simulink model "SEPIC_PV_system_MPPT_Alogrithms_BATTERY"  (R2025a)
settings: Solver=FixedStepAuto  StartTime=0.0  StopTime=1  FixedStep=1e-7  RelTol=1e-3
undefined symbols (not defined in the file): Ion, Lithium, sigbuilder_block
libraries: spsSeriesRLCBranchLib x6, spsCurrentMeasurementLib x5, spsVoltageMeasurementLib x3, spsGroundLib x2, spsBatteryLib x1, spsDiodeLib x1, spsMosfetLib x1, spsPVArrayLib x1, simulink x1, simulink_extras x1, sps_lib x1
settings Model: Creator=gamezebra  LastModifiedBy=gamezebra

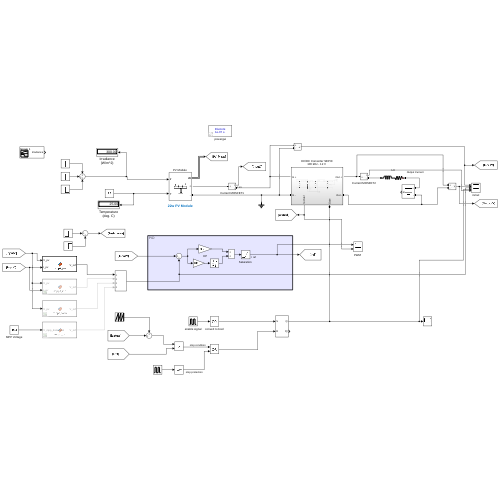
[thumbnail: Simulink's stored preview of the top-level diagram]
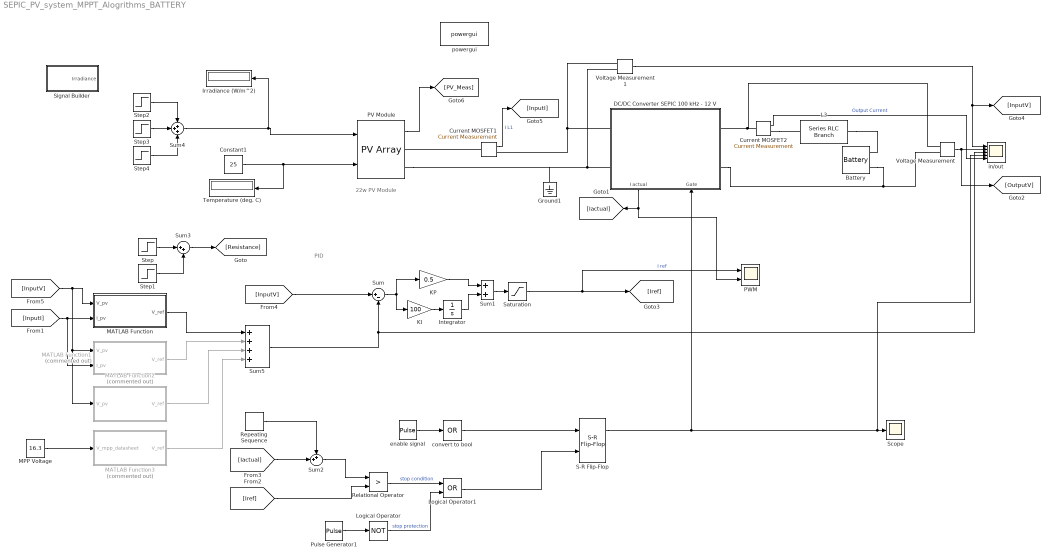
== system SEPIC_PV_system_MPPT_Alogrithms_BATTERY ==
  note: PID
  note: 22w PV Module
  Battery : spsBatteryLib/Battery  BatType=Lithium-Ion  NomV=10.8  NomQ=1  SOC=3  Batt_Tr=30  PresetModel=on  MaxQ=1  MinV=8.1  FullV=12.5711  Dis_rate=0.43478  R=0.108  Normal_OP=0.90435  expZone="[11.6682    0.0491304]"
  Constant1 : Constant  Value=25
  Current MOSFET1 : spsCurrentMeasurementLib/Current Measurement  PhasorSimulation=off  OutputType=Complex  PSBequivalent=0
  Current MOSFET2 : spsCurrentMeasurementLib/Current Measurement  PhasorSimulation=off  OutputType=Complex  PSBequivalent=0
  "DC/DC Converter SEPIC 100 kHz - 12 V " : Subsystem
      settings: PortSchema="{\"entries\":[{\"content\":{\"sides\":[{\"content\":{\"connectorIds\":[\"LConn1\",\"LConn2\"]},\"type\":\"ConnectorPlacement.EquallySpacedRectSide\",\"uuid\":\"91feb529-5820-4edf-8d0e-1c637fed9421\"},{\"content\":{\"connectorIds\":[\"RConn1\",\"RConn2\"],\"side\":\"RIGHT\"},\"type\":\"ConnectorPlacement.EquallySpacedRectSide\",\"uuid\":\"b4099113-c0ef-4c50-8083-88b14b98cc04\"},{\"content\":{\"side\":\"TOP\"},\"type\":\"ConnectorPlacement.EquallySpacedRectSide\",\"uuid\":\"250c6351-2de3-43d7-b6c9-3c3ed0452184\"},{\"content\":{\"connectorIds\":[\"Out1\",\"In1\"],\"side\":\"BOTTOM\"},\"type\":\"ConnectorPlacement.EquallySpacedRectSide\",\"uuid\":\"484af620-bbf2-4328-991e-a08b15b59058\"}]},\"type\":\"ConnectorPlacement.EquallySpacedConnector\",\"uuid\":\"7041a545-1967-46d5-8643-e26f6c990daf\"}],\"packageUris\":[\"http://schema.mathworks.com/mf0/Connector/R2020b\"],\"version\":\"1.0\"}"
  Ground1 : spsGroundLib/Ground  LConnTagsString=a
  Integrator : Integrator  LimitOutput=on  UpperSaturationLimit=8  LowerSaturationLimit=0
  Irradiance (W/m^2) : Display
      settings: Format=bank  Decimation=1000
  KI : Gain  Gain=100
  KP : Gain  Gain=0.5
  L3 : spsSeriesRLCBranchLib/Series RLC Branch  LConnTagsString=__new0  RConnTagsString=__new0  BranchType=RL  Resistance=0.1  Inductance=5e-6  SetiL0=off  InitialCurrent=0  Capacitance=1e-6  Setx0=off  InitialVoltage=0  Measurements=None
  Logical Operator : Logic  Operator=NOT  AllPortsSameDT=off  OutDataTypeStr=boolean
  Logical Operator1 : Logic  Operator=OR  AllPortsSameDT=off  OutDataTypeStr=boolean
  MATLAB Function : MATLAB Function  TreatAsAtomicUnit=on
  MATLAB Function1 : MATLAB Function  Commented=on  TreatAsAtomicUnit=on
  MATLAB Function2 : MATLAB Function  Commented=on  TreatAsAtomicUnit=on
  MATLAB Function3 : MATLAB Function  Commented=on  TreatAsAtomicUnit=on
  MPP Voltage : Constant  Value=16.3
  "PV Module " : spsPVArrayLib/PV Array  Npar=1  Nser=1  PlotType=one module @ 25 deg.C & specified irradiances  S_vec="[ 1000  500  200 ]"  Temp_C_vec=25  ModuleName=User-defined  PlotWhenSelected=off  Pm=21.6138  Ncell=30  Voc=17.76  Isc=1.5  Vm=16.3  Im=1.326  beta_Voc_pc=-0.37  alpha_Isc_pc=0.07  beta_Voc=-0.065712  alpha_Isc=0.00105  IL=1.5  I0=2.021e-11  nI=1.0007  Rsh=187.3567  Rs=0.40236  RobustModel=off  RobustCellTemperature=313.3991  BAL=on  Tc=1e-6  Tfilter=5e-5
  "PWM " : Scope  NumInputPorts=2
      settings: Title=PWM  ActiveDisplayYMinimum=3.3246670438564179  ActiveDisplayYMaximum=8.2208811739016561  YLabel=Amplitudo
  Pulse Generator1 : DiscretePulseGenerator  PulseType=Time based  Period=10e-6  PulseWidth=90
  Relational Operator : RelationalOperator  Operator=>  OutDataTypeStr=boolean  RndMeth=Simplest  InputSameDT=off
  Repeating Sequence : simulink/Sources/Repeating Sequence  rep_seq_t=[0 10e-6]  rep_seq_y=[0 2]
  S-R Flip-Flop : simulink_extras/Flip Flops/S-R Flip-Flop  initial_condition=0
  "Saturation " : Saturate  UpperLimit=8  LowerLimit=0
  Scope : Scope
      settings: ActiveDisplayYMinimum=-0.12499999999999997  ActiveDisplayYMaximum=1.125  DataLoggingVariableName=ScopeData2
  Signal Builder : Subsystem  Tag=STV Subsys  LoadFcn=sigbuilder_block('load');  StartFcn=sigbuilder_block('start');  StopFcn=sigbuilder_block('stop');  ClipboardFcn=sigbuilder_block('clipboard');  mask(Sigbuilder block){tuvar=[0:10]}
      mask help: Simulink:masks:SigbuilderBlock_MD
      mask init:
      | if ~strcmp(get_param(bdroot(gcbh),'SimulationStatus'),'stopped') tuvar = sigbuilder_block('maskInit'); end
      settings: CopyFcn=sigbuilder_block('copy');  DeleteFcn=sigbuilder_block('delete');  ModelCloseFcn=sigbuilder_block('modelClose');  PreSaveFcn=sigbuilder_block('preSave');  PauseFcn=sigbuilder_block('pause');  ContinueFcn=sigbuilder_block('continue');  NameChangeFcn=sigbuilder_block('namechange');  OpenFcn=sigbuilder_block('open',[237.75 162.75 783 471.75 ]);  CloseFcn=sigbuilder_block('close');
      mask Display: plot(0, 0, 100, 100,[2, 2, 32, 32, 2], [68, 8, 8, 68, 68],[32, 2], [38, 38], [32, 19, 2],[53, 60, 44], [32, 17, 17, 2],[16, 16, 31, 31]);txt = getActiveGroup(gcbh);text(2, 100, txt,'verticalAlignment', 'top');
  Step : Step  Time=0  After=0  SampleTime=0
  Step1 : Step  Time=0  After=30  SampleTime=0
  Step2 : Step  Time=0.3  Before=1000  After=800  SampleTime=0
  Step3 : Step  Time=0.5  After=-300  SampleTime=0
  Step4 : Step  Time=0.7  After=-200  SampleTime=0
  Sum : Sum  Inputs=|+-
  Sum1 : Sum
  Sum2 : Sum  Inputs=++|
  Sum3 : Sum  Inputs=|++
  Sum4 : Sum  Inputs=+++
  Sum5 : Sum  Inputs=++++
  Temperature (deg. C) : Display
      settings: Format=bank  Decimation=1000
  Voltage Measurement : spsVoltageMeasurementLib/Voltage Measurement  PhasorSimulation=off  OutputType=Complex  PSBequivalent=0
  Voltage Measurement1 : spsVoltageMeasurementLib/Voltage Measurement  PhasorSimulation=off  OutputType=Complex  PSBequivalent=0
  convert to bool : Logic  Operator=OR  Inputs=1  AllPortsSameDT=off  OutDataTypeStr=boolean
  enable signal : DiscretePulseGenerator  PulseType=Time based  Period=10e-6  PulseWidth=5
  in/out : Scope  NumInputPorts=5
      settings: Title=PWM  ActiveDisplayYMinimum=-3.0785426285562241  ActiveDisplayYMaximum=22.486425523480442  YLabel=Amplitudo  DataLoggingVariableName=ScopeData3
  powergui : sps_lib/powergui  Priority=1  SimulationMode=Discrete  SampleTime=1e-7  frequency=60  Iterations=50  frequencyindice=0  Pbase=100e6  ErrMax=1e-4  UnitsV=kV  UnitsW=MW  buscounter=0  FunctionMessages=off  echomessages=off  EnableUseOfTLC=off  CurrentSourceSwitches=off  DisableSnubberDevices=off  DisableRonSwitches=off  DisableVfSwitches=off  DisplayEquations=off  AutomaticDiscreteSolvers=off  SolverType=Tustin/Backward Euler (TBE)  Interpol=off  ExternalGateDelay=off  methode=off  Ts=100  x0status=blocks  SPID=on  SwTol=0  HookPort=off  NonlinearTolerance=1e-4  nMaxIteration=100  ContinueOnMaxIteration=off  RestoreLinks=warning  ResistiveCurrentMeasurement=off  Frange=[0:2:500]  Ylog=off  Xlog=on  ShowGrid=off  save=off  variable=ZData  structure=0  ZoomFFT=off  StartTime=0.0  cycles=1  DisplayStyle=1  fundamental=60  FreqAxis=off  MaxFrequency=1000  frequencyindicesteady=1  RmsSteady=1  display=off
  wires:
  Voltage Measurement1/1 -> in/out/1, [InputV]
  Voltage Measurement/1 -> [OutputV], in/out/2
  Step/1 -> Sum3/1
  Sum1/1 -> "Saturation "/1
  KI/1 -> Integrator/1
  Integrator/1 -> Sum1/2
  KP/1 -> Sum1/1
  Sum/1 -> KI/1, KP/1
  "Saturation "/1 -> "PWM "/1, [Iref]  "I ref"
  [InputV] -> Sum/1
  S-R Flip-Flop/1 -> in/out/4, Scope/1, "DC/DC Converter SEPIC 100 kHz - 12 V "/1(Gate)
  [Iactual] -> Sum2/2
  Pulse Generator1/1 -> Logical Operator/1
  Relational Operator/1 -> Logical Operator1/1  "stop condition"
  Logical Operator/1 -> Logical Operator1/2  "stop protection"
  "DC/DC Converter SEPIC 100 kHz - 12 V "/1(I actual) -> "PWM "/2, [Iactual]
  [Iref] -> Relational Operator/2
  Logical Operator1/1 -> S-R Flip-Flop/2
  enable signal/1 -> convert to bool/1
  convert to bool/1 -> S-R Flip-Flop/1
  Repeating Sequence/1 -> Sum2/1
  Sum2/1 -> Relational Operator/1
  Step1/1 -> Sum3/2
  Sum3/1 -> [Resistance]
  "PV Module "/1 -> [PV_Meas]
  Constant1/1 -> "PV Module "/2, Temperature (deg. C)/1
  Step3/1 -> Sum4/2
  Step2/1 -> Sum4/1
  Step4/1 -> Sum4/3
  Current MOSFET1/1 -> [InputI]  "I L1"
  [InputI] -> MATLAB Function1/2(I_pv), MATLAB Function/2(I_pv)
  [InputV] -> MATLAB Function2/1(V_pv), MATLAB Function1/1(V_pv), MATLAB Function/1(V_pv)
  MATLAB Function/1(V_ref) -> Sum5/1
  Sum4/1 -> Irradiance (W/m^2)/1, "PV Module "/1
  Sum5/1 -> in/out/3, Sum/2
  MATLAB Function1/1(V_ref) -> Sum5/2
  MATLAB Function2/1(V_ref) -> Sum5/3
  MATLAB Function3/1(V_ref) -> Sum5/4
  MPP Voltage/1 -> MATLAB Function3/1(V_mpp_datasheet)
  Current MOSFET2/1 -> in/out/5  "Output Current"
  connections:
  Voltage Measurement1/LConn1 -- Current MOSFET1/RConn1 -- "DC/DC Converter SEPIC 100 kHz - 12 V "/LConn1
  Current MOSFET2/RConn1 -- L3/RConn1
  "DC/DC Converter SEPIC 100 kHz - 12 V "/RConn2 -- Battery/LConn2 -- Voltage Measurement/LConn2
  "DC/DC Converter SEPIC 100 kHz - 12 V "/LConn2 -- Voltage Measurement1/LConn2 -- "PV Module "/RConn2 -- Ground1/LConn1
  Current MOSFET1/LConn1 -- "PV Module "/RConn1
  Voltage Measurement/LConn1 -- Current MOSFET2/LConn1 -- "DC/DC Converter SEPIC 100 kHz - 12 V "/RConn1
  L3/LConn1 -- Battery/LConn1

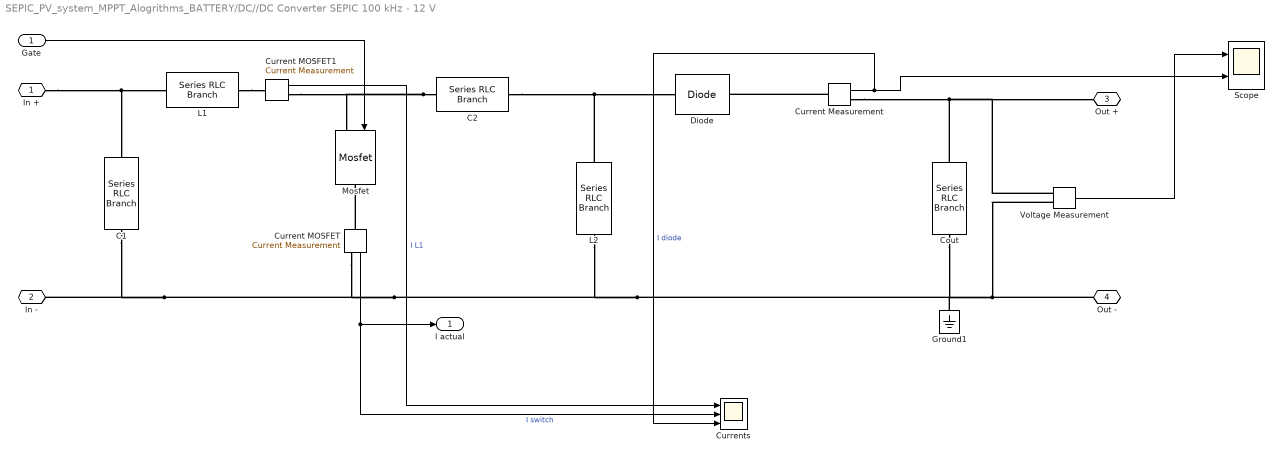
== system SEPIC_PV_system_MPPT_Alogrithms_BATTERY/DC//DC Converter SEPIC 100 kHz - 12 V  ==
  Gate : Inport
  C1 : spsSeriesRLCBranchLib/Series RLC Branch  LConnTagsString=__new0  RConnTagsString=__new0  BranchType=RC  Resistance=0.01  Inductance=1e-3  SetiL0=off  InitialCurrent=0  Capacitance=0.00001  Setx0=on  InitialVoltage=18  Measurements=None
  C2 : spsSeriesRLCBranchLib/Series RLC Branch  LConnTagsString=__new0  RConnTagsString=__new0  BranchType=C  Resistance=1  Inductance=1e-3  SetiL0=off  InitialCurrent=0  Capacitance=0.00001  Setx0=off  InitialVoltage=0  Measurements=None
  Cout : spsSeriesRLCBranchLib/Series RLC Branch  LConnTagsString=__new0  RConnTagsString=__new0  BranchType=RC  Resistance=0.01  Inductance=16.8e-3  SetiL0=off  InitialCurrent=0  Capacitance=0.0001  Setx0=on  InitialVoltage=11.63  Measurements=None
  Current MOSFET : spsCurrentMeasurementLib/Current Measurement  PhasorSimulation=off  OutputType=Complex  PSBequivalent=0
  Current MOSFET1 : spsCurrentMeasurementLib/Current Measurement  PhasorSimulation=off  OutputType=Complex  PSBequivalent=0
  "Current Measurement " : spsCurrentMeasurementLib/Current Measurement  PhasorSimulation=off  OutputType=Complex  PSBequivalent=0
  Currents : Scope  NumInputPorts=3
      settings: ActiveDisplayYMinimum=-2.4566036573506662  ActiveDisplayYMaximum=3.5153800209257291  DataLoggingVariableName=ScopeData4
  "Diode " : spsDiodeLib/Diode  Ron=0.001  Lon=0  Vf=0.5  IC=0  UseSnubber=0  Rs=500  Cs=250e-9  Measurements=off
  Ground1 : spsGroundLib/Ground  LConnTagsString=a
  L1 : spsSeriesRLCBranchLib/Series RLC Branch  LConnTagsString=__new0  RConnTagsString=__new0  BranchType=RL  Resistance=0.2  Inductance=0.0002  SetiL0=off  InitialCurrent=0  Capacitance=1e-6  Setx0=off  InitialVoltage=0  Measurements=None
  L2 : spsSeriesRLCBranchLib/Series RLC Branch  LConnTagsString=__new0  RConnTagsString=__new0  BranchType=RL  Resistance=0.2  Inductance=0.0002  SetiL0=off  InitialCurrent=0  Capacitance=1e-6  Setx0=off  InitialVoltage=0  Measurements=None
  Mosfet : spsMosfetLib/Mosfet  Ron=0.1  Lon=0  Rd=0.01  Vfd=0  IC=0  Rs=1e5  Cs=inf  Measurements=off
  Scope : Scope  NumInputPorts=2
      settings: Title=Tegangan Keluaran Konverter SEPIC  ActiveDisplayYMinimum=-151.86738214367281  ActiveDisplayYMaximum=1366.8064463408562  YLabel=Tegangan (Volts)
  "Voltage Measurement " : spsVoltageMeasurementLib/Voltage Measurement  PhasorSimulation=off  OutputType=Complex  PSBequivalent=0
  In + : PMIOPort  Side=Left
  In - : PMIOPort  Port=2  Side=Left
  Out + : PMIOPort  Port=3  Side=Right
  Out - : PMIOPort  Port=4  Side=Right
  I actual : Outport
  wires:
  Gate/1 -> Mosfet/1
  "Current Measurement "/1 -> Currents/3, Scope/2  "I diode"
  "Voltage Measurement "/1 -> Scope/1
  Current MOSFET/1 -> Currents/2, I actual/1  "I switch"
  Current MOSFET1/1 -> Currents/1  "I L1"
  connections:
  Out -/RConn1 -- Cout/RConn1 -- Ground1/LConn1 -- L2/RConn1 -- C1/RConn1 -- In -/RConn1 -- Current MOSFET/RConn1 -- "Voltage Measurement "/LConn2
  C2/LConn1 -- Current MOSFET1/RConn1 -- Mosfet/LConn1
  C2/RConn1 -- L2/LConn1 -- "Diode "/LConn1
  In +/RConn1 -- C1/LConn1 -- L1/LConn1
  "Current Measurement "/LConn1 -- "Diode "/RConn1
  Current MOSFET/LConn1 -- Mosfet/RConn1
  L1/RConn1 -- Current MOSFET1/LConn1
  Cout/LConn1 -- Out +/RConn1 -- "Voltage Measurement "/LConn1 -- "Current Measurement "/RConn1

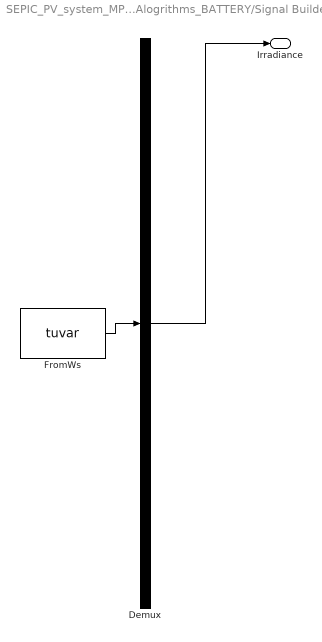
== system SEPIC_PV_system_MPPT_Alogrithms_BATTERY/Signal Builder ==
  Demux : Demux  Tag=STV Demux  Outputs=1
      settings: DisplayOption=none
  FromWs : FromWorkspace  Tag=STV FromWs  VariableName=tuvar
      SigBuilderData=|
      | common.afterFinalStr = 'Extrapolate'
      | common.sampleTime = 0
      | dataSet.timeRange = [0 2]
      | dataSet.name = 'Group 1'
      | sbobj.Groups.Name = 'Group 1'
      | sbobj.Groups.Signals.Name = 'Irradiance'
      | sbobj.Groups.Signals.XData = [0 0.48 0.48 0.52 0.98 0.98 1.235 1.48 1.66 1.66 2]
      | sbobj.Groups.Signals.YData = [502 502 500 802 802 801 538 626 927 928 926]
      | sbobj.Groups.TimeRange = [0 2]
  Irradiance : Outport  Tag=STV Outport
  wires:
  Demux/1 -> Irradiance/1
  FromWs/1 -> Demux/1

== matlab function SEPIC_PV_system_MPPT_Alogrithms_BATTERY/MATLAB Function ==
  data: V_pv input; V_ref output; I_pv input
function V_ref = mppt_po(V_pv, I_pv)
    % Perturb and Observe
    % Дефиниране на постоянни променливи (пазят състоянието между стъпките)
    persistent P_prev V_prev V_ref_prev counter
    
    % --- НАСТРОЙКИ НА АЛГОРИТЪМА ---
    delta_V = 0.5;          % Стъпка на промяна на напрежението (във Волтове)
    V_min = 12.0;           % Долна граница (предпазва от Latch-up и късо съединение)
    V_max = 19.0;           % Горна граница (близо до Voc на панела)
    MPPT_Period = 250000;   % На колко симулационни стъпки да се изпълнява алгоритъмът
    
    % Инициализация при първо стартиране на симулацията (t=0)
    if isempty(counter)
        P_prev = 0;
        V_prev = 0;
        V_ref_prev = 18.0;  % Стартираме безопасно близо до Open-Circuit
        counter = 0;
    end
    
    % Увеличаваме брояча при всяка стъпка на симулатора
    counter = counter + 1;
    
    % По подразбиране задържаме старото задание
    V_ref = V_ref_prev; 
    
    % Изпълняваме P&O логиката само когато броячът прелее
    if counter >= MPPT_Period
        % Изчисляваме текущата мощност
        P_pv = V_pv * I_pv;
        
        % Изчисляваме разликите
        dP = P_pv - P_prev;
        dV = V_pv - V_prev;
        
        % Perturb & Observe логика
        if dP ~= 0
            if dP > 0
                if dV > 0
                    V_ref_new = V_ref_prev + delta_V;
                else
                    V_ref_new = V_ref_prev - delta_V;
                end
            else
                if dV > 0
                    V_ref_new = V_ref_prev - delta_V;
                else
                    V_ref_new = V_ref_prev + delta_V;
                end
            end
            
            % Прилагаме защитните лимити
            if V_ref_new > V_max
                V_ref_new = V_max;
            elseif V_ref_new < V_min
                V_ref_new = V_min;
            end
            
            % Обновяваме изхода
            V_ref = V_ref_new;
            V_ref_prev = V_ref_new;
        end
        
        % Запаметяваме текущите стойности за следващия цикъл
        P_prev = P_pv;
        V_prev = V_pv;
        counter = 0; % Рестартираме брояча
    end
end

== matlab function SEPIC_PV_system_MPPT_Alogrithms_BATTERY/MATLAB Function2 ==
  data: V_pv input; V_ref output
function V_ref = mppt_focv(V_pv)
    % fractional open circuit voltage
    % Пазим състоянието и променливите между симулационните стъпки
    persistent state counter V_oc_measured V_ref_out
    
    % --- НАСТРОЙКИ НА АЛГОРИТЪМА ---
    k_focv = 0.80;          % Фиксиран процент (80% от Voc)
    V_max = 25.0;           % Изкуствено високо задание за форсиране на празен ход
    
    % Времеви настройки (в брой симулационни стъпки при 1e-7 s)
    T_mppt = 500000;        % Време за нормална работа (напр. 50 ms)
    T_settle = 100000;       % Време за разтоварване и измерване на Voc (напр. 1 ms)
    
    % Инициализация при t=0
    if isempty(state)
        state = 1;          % Стартираме директно в режим на измерване
        counter = 0;
        V_oc_measured = 20.0; 
        V_ref_out = V_max;  
    end
    
    % Увеличаваме брояча при всяка стъпка
    counter = counter + 1;
    
    if state == 0 
        % ----------------------------------------------------
        % СЪСТОЯНИЕ 0: Нормална работа (MPPT Tracking)
        % ----------------------------------------------------
        V_ref_out = k_focv * V_oc_measured;
        
        if counter >= T_mppt
            % Времето за работа изтече, преминаваме към измерване
            state = 1; 
            counter = 0;
            V_ref_out = V_max; % Форсираме ПИ регулатора към 0А ток
        end
        
    elseif state == 1 
        % ----------------------------------------------------
        % СЪСТОЯНИЕ 1: Изчакване и Измерване (Open-Circuit)
        % ----------------------------------------------------
        V_ref_out = V_max; 
        
        if counter >= T_settle
            % Панелът е разтоварен, запаметяваме реалното Voc
            V_oc_measured = V_pv;
            
            % Връщаме се в нормален режим с новото изчислено задание
            state = 0;
            counter = 0;
            V_ref_out = k_focv * V_oc_measured;
        end
    end
    
    % Подаваме сигнала към изхода на блока
    V_ref = V_ref_out;
end

== matlab function SEPIC_PV_system_MPPT_Alogrithms_BATTERY/MATLAB Function3 ==
  data: V_mpp_datasheet input; V_ref output
function V_ref = mppt_cv(V_mpp_datasheet)
    % Constant Voltage (CV) MPPT 
    % Директно прехвърля статичното задание от дейташийта.
    
    V_ref = V_mpp_datasheet;
end

== matlab function SEPIC_PV_system_MPPT_Alogrithms_BATTERY/MATLAB Function1 ==
  data: V_pv input; V_ref output; I_pv input
function V_ref = mppt_inc(V_pv, I_pv)
    % incremental conductance
    persistent I_prev V_prev V_ref_prev counter
    
    % --- НАСТРОЙКИ НА АЛГОРИТЪМА ---
    delta_V = 0.5;          % Стъпка на промяна на напрежението
    V_min = 12.0;           % Долна граница
    V_max = 19.0;           % Горна граница
    MPPT_Period = 100000;   % Период на изпълнение (брой симулационни стъпки)
    epsilon = 0.05;         % Толеранс за сравняване с нула (много важно!)
    
    % Инициализация
    if isempty(counter)
        I_prev = 0;
        V_prev = 0;
        V_ref_prev = 18.0;  % Безопасен старт
        counter = 0;
    end
    
    counter = counter + 1;
    V_ref = V_ref_prev; 
    
    if counter >= MPPT_Period
        dV = V_pv - V_prev;
        dI = I_pv - I_prev;
        
        if abs(dV) < epsilon  % Ако напрежението не се е променило (dV = 0)
            if dI > epsilon
                V_ref_new = V_ref_prev + delta_V;
            elseif dI < -epsilon
                V_ref_new = V_ref_prev - delta_V;
            else
                V_ref_new = V_ref_prev; % dV = 0 и dI = 0 (няма промяна)
            end
        else
            % Изчисляване на двете проводимости
            inc_cond = dI / dV;
            inst_cond = -I_pv / V_pv;
            
            % Сравняване с толеранс
            if abs(inc_cond - inst_cond) < epsilon
                V_ref_new = V_ref_prev; % На върха сме! Спираме промяната.
            elseif inc_cond > inst_cond
                V_ref_new = V_ref_prev + delta_V; % Вляво от върха, увеличаваме V
            else
                V_ref_new = V_ref_prev - delta_V; % Вдясно от върха, намаляваме V
            end
        end
        
        % Защитни лимити
        if V_ref_new > V_max
            V_ref_new = V_max;
        elseif V_ref_new < V_min
            V_ref_new = V_min;
        end
        
        V_ref = V_ref_new;
        V_ref_prev = V_ref_new;
        
        % Запаметяване за следващия цикъл
        I_prev = I_pv;
        V_prev = V_pv;
        counter = 0;
    end
end
